simulink model "HexaMotor_System_Identification_V02_250Hz"  (R2024b)
settings: Solver=FixedStepDiscrete  StartTime=0.0  StopTime=2  FixedStep=0.004  RelTol=1e-3  EnableMultiTasking=on
libraries: arduinolib x3, arduinosensorlib x1, eeGeneralControl x1, simulink x1
settings Model: ExtModeTrigDuration=2  Creator=bkhusain  LastModifiedBy=arkad
settings SolverCC: AlgebraicLoopSolver=TrustRegion  AutoInsertRateTranBlk=on
settings DataIOCC: SaveOutput=off  DSMLogging=off  SaveTime=off  ReturnWorkspaceOutputs=off
settings OptimizationCC: EnhancedBackFolding=on  PassReuseOutputArgsThreshold=0  MaxStackSize=64  OptimizeBlockOrder=speed  DifferentSizesBufferReuse=on  OptimizationCustomize=off
settings DebuggingCC: ParameterOverflowMsg=none  ParameterUnderflowMsg=error  ParameterPrecisionLossMsg=none  ParameterTunabilityLossMsg=error  UnconnectedInputMsg=warning  UnconnectedOutputMsg=warning  UnconnectedLineMsg=warning
settings HardwareCC: ProdBitPerPointer=32  ProdBitPerSizeT=32  ProdBitPerPtrDiffT=32  ProdLargestAtomicInteger=Long  ProdLargestAtomicFloat=Double  ProdWordSize=32  ProdHWDeviceType=ARM Compatible->ARM Cortex
settings ModelReferenceCC: EnableRefExpFcnMdlSchedulingChecks=on
settings SFSimCC: MATLABDynamicMemAlloc=off
settings RTWCC: Description=Embedded Coder  SystemTargetFile=ert.tlc  HardwareBoard=Arduino MKRZero  TemplateMakefile=ert_default_tmf  Toolchain=Arduino ARM  BuildConfiguration=Faster Runs  GPUComputeCapability=3.5  DLArmComputeVersion=19.05
settings CodeAppCC: ForceParamTrailComments=on  OperatorAnnotations=on
settings ERTTargetCC: ERTCustomFileBanners=off  SupportContinuousTime=on  SupportNonInlinedSFcns=on  RemoveResetFunc=off  SupportVariableSizeSignals=on  ModelStepFunctionPrototypeControlCompliant=off  ExtModeTransport=3  ExtModeStaticAlloc=on  ExtModeAutomaticAllocSize=off  ExtModeStaticAllocSize=8192  ExtModeMexFile=ext_xcp  ExtModeIntrfLevel=Level2 - Open  InlinedParameterPlacement=Hierarchical  DynamicArrayContainerType=coder::array

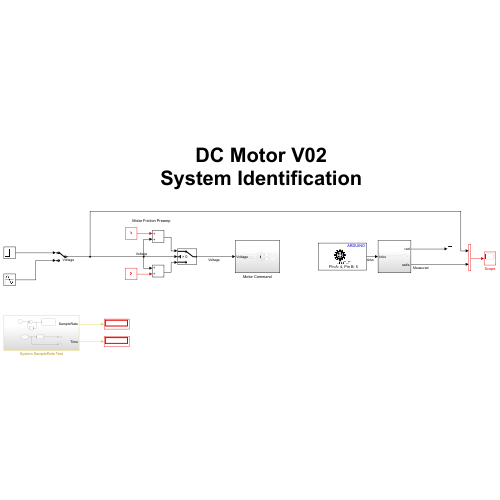
[thumbnail: Simulink's stored preview of the top-level diagram]
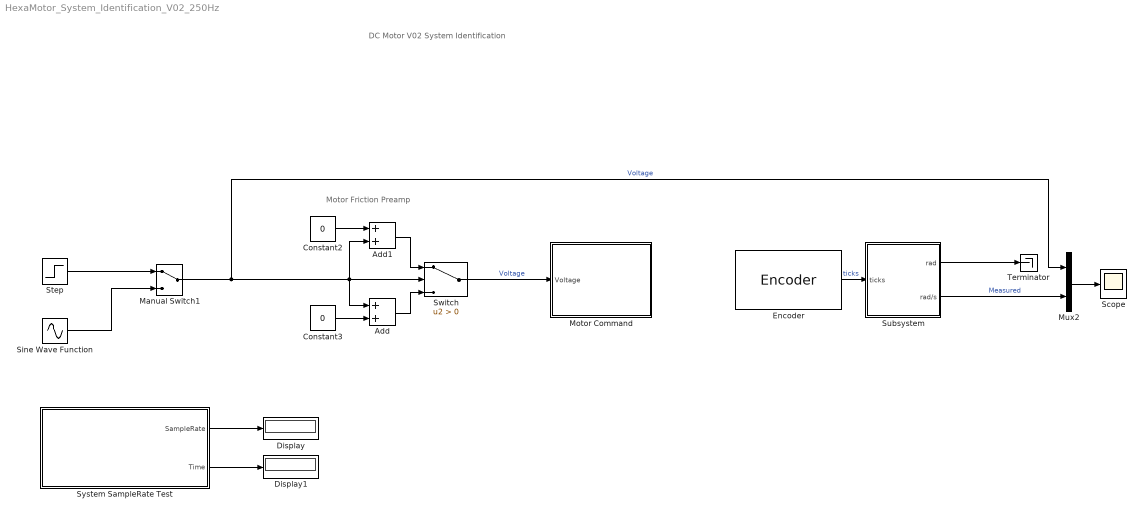
== system HexaMotor_System_Identification_V02_250Hz ==
  note: DC Motor V02
      | System Identification
  note: Motor Friction Preamp
  Add : Sum
  Add1 : Sum
  Constant2 : Constant  Value=0  SampleTime=-1
  Constant3 : Constant  Value=0  SampleTime=-1
  Display : Display
  Display1 : Display
  Encoder : arduinosensorlib/Encoder  InputA=4  InputB=5  Mode=No reset  SampleTime=-1
      settings: SourceProductName=Sensors
  Manual Switch1 : ManualSwitch
  Motor Command : Subsystem
  Mux2 : Mux  Inputs=2
  Scope : Scope
  Sine Wave Function : Sin  Amplitude=7
  Step : Step  After=7
  Subsystem : Subsystem
  Switch : Switch  Criteria=u2 > Threshold  SaturateOnIntegerOverflow=off  InputSameDT=off
  System SampleRate Test : Subsystem
  Terminator : Terminator
  wires:
  System SampleRate Test/1(SampleRate) -> Display/1
  System SampleRate Test/2(Time) -> Display1/1
  Mux2/1 -> Scope/1
  Step/1 -> Manual Switch1/1
  Sine Wave Function/1 -> Manual Switch1/2
  Manual Switch1/1 -> Mux2/1, Add1/2, Switch/2, Add/1  "Voltage"
  Add/1 -> Switch/3
  Switch/1 -> Motor Command/1(Voltage)  "Voltage"
  Constant2/1 -> Add1/1
  Constant3/1 -> Add/2
  Add1/1 -> Switch/1
  Encoder/1 -> Subsystem/1(ticks)  "ticks"
  Subsystem/1(rad) -> Terminator/1
  Subsystem/2(rad/s) -> Mux2/2  "Measured"

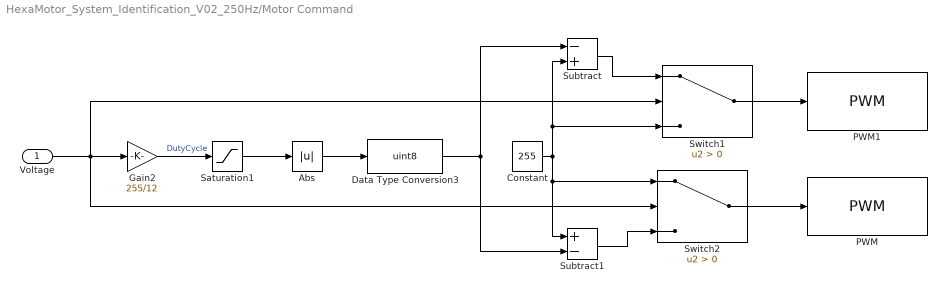
== system HexaMotor_System_Identification_V02_250Hz/Motor Command ==
  Voltage : Inport
  Abs : Abs  SaturateOnIntegerOverflow=off
  Constant : Constant  Value=255  OutDataTypeStr=uint8  SampleTime=-1
  Data Type Conversion3 : DataTypeConversion  OutDataTypeStr=uint8  SaturateOnIntegerOverflow=off  RndMeth=Floor
  Gain2 : Gain  Gain=255/12
  PWM : arduinolib/PWM  pinNumber=2  frequencyType=Specify  desiredFrequency=5000  achievableFrequency=5000
      settings: LibrarySourceBlock=gizmoLibrary/Arduino Utilities/PWM  SourceProductName=Common
  PWM1 : arduinolib/PWM  pinNumber=3  frequencyType=Specify  desiredFrequency=5000  achievableFrequency=5000
      settings: LibrarySourceBlock=gizmoLibrary/Arduino Utilities/PWM  SourceProductName=Common
  Saturation1 : Saturate  UpperLimit=255  LowerLimit=-255
  Subtract : Sum  Inputs=-+
  Subtract1 : Sum  Inputs=+-
  Switch1 : Switch  Criteria=u2 > Threshold  OutDataTypeStr=uint8  SaturateOnIntegerOverflow=off  InputSameDT=off
  Switch2 : Switch  Criteria=u2 > Threshold  OutDataTypeStr=uint8  SaturateOnIntegerOverflow=off  InputSameDT=off
  wires:
  Voltage/1 -> Switch2/2, Switch1/2, Gain2/1
  Abs/1 -> Data Type Conversion3/1
  Subtract/1 -> Switch1/1
  Gain2/1 -> Saturation1/1  "DutyCycle"
  Subtract1/1 -> Switch2/3
  Constant/1 -> Switch1/3, Subtract/2, Subtract1/1, Switch2/1
  Data Type Conversion3/1 -> Subtract/1, Subtract1/2
  Saturation1/1 -> Abs/1
  Switch1/1 -> PWM1/1
  Switch2/1 -> PWM/1

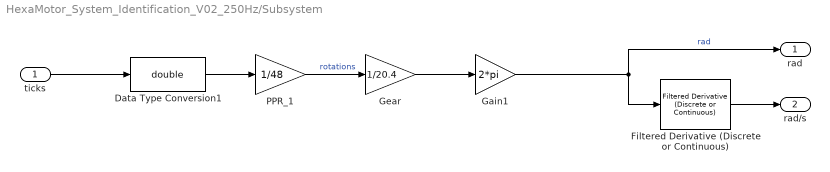
== system HexaMotor_System_Identification_V02_250Hz/Subsystem ==
  ticks : Inport
  Data Type Conversion1 : DataTypeConversion  OutDataTypeStr=double  SaturateOnIntegerOverflow=off  RndMeth=Floor
  Filtered Derivative (Discrete or Continuous) : eeGeneralControl/Filtered Derivative (Discrete or Continuous)  K=1  T=0.05  B=inf  A=-inf  minRatio=10  init_option=Inherited from block input  x0=0  Ts=-1
      settings: LibrarySourceBlock=|
      | ee_sl_lib/General Control/Filtered Derivative
      | (Discrete or Continuous)
  Gain1 : Gain  Gain=2*pi
  Gear : Gain  Gain=1/20.4
  PPR_1 : Gain  Gain=1/48
  rad : Outport
  rad/s : Outport  Port=2
  wires:
  PPR_1/1 -> Gear/1  "rotations"
  Data Type Conversion1/1 -> PPR_1/1
  ticks/1 -> Data Type Conversion1/1
  Gear/1 -> Gain1/1
  Gain1/1 -> rad/1, Filtered Derivative (Discrete or Continuous)/1  "rad"
  Filtered Derivative (Discrete or Continuous)/1 -> rad/s/1

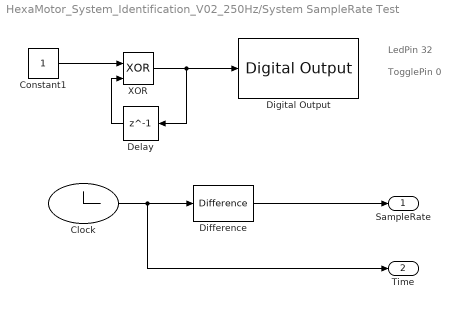
== system HexaMotor_System_Identification_V02_250Hz/System SampleRate Test ==
  note: LedPin 32
  note: TogglePin 0
  Clock : Clock
      settings: Decimation=3
  Constant1 : Constant  SampleTime=-1
  Delay : Delay  DelayLength=1  InitialCondition=0
  Difference : simulink/Quick Insert/Discrete/Difference  ICPrevInput=0.0  OutMin=[]  OutMax=[]  OutDataType=fixdt(1, 16)  OutScaling=2^-10  DoSatur=off
  Digital Output : arduinolib/Digital Output  pinNumber=32  Direction=output  blockPlatform=arduino
      settings: SourceProductName=Common
  XOR : Logic  Operator=XOR  IconShape=distinctive  AllPortsSameDT=off  OutDataTypeStr=boolean
  SampleRate : Outport
  Time : Outport  Port=2
  wires:
  XOR/1 -> Delay/1, Digital Output/1
  Constant1/1 -> XOR/1
  Delay/1 -> XOR/2
  Clock/1 -> Time/1, Difference/1
  Difference/1 -> SampleRate/1
